simulink model "pardosealasim"  (R2023b)
settings: Solver=VariableStepAuto  StartTime=0.0  StopTime=12000  RelTol=1e-3
values from neighbouring files (symbols this model uses):
  A = [-(1/Tp) 1/Tp; Kp/(Kc*Tc) -((1+(Kp/Kc))/Tc)]    [pardoseala.m]
  B = [KE/(Kp*Tp) 0;0 1/Tc]    [pardoseala.m]
  C = [1 0;0 1]    [pardoseala.m]
  D = [0 0;0 0]    [pardoseala.m]
  Kc = 125    [pardoseala.m]
  KE = 1000    [pardoseala.m]
  Kp = 500    [pardoseala.m]
  Tc = 300    [pardoseala.m]
  Tp = 60    [pardoseala.m]
settings Model: Creator=Bianca  LastModifiedBy=Bianca

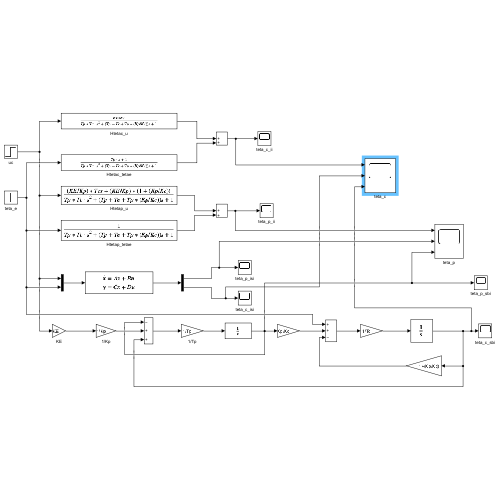
[thumbnail: Simulink's stored preview of the top-level diagram]
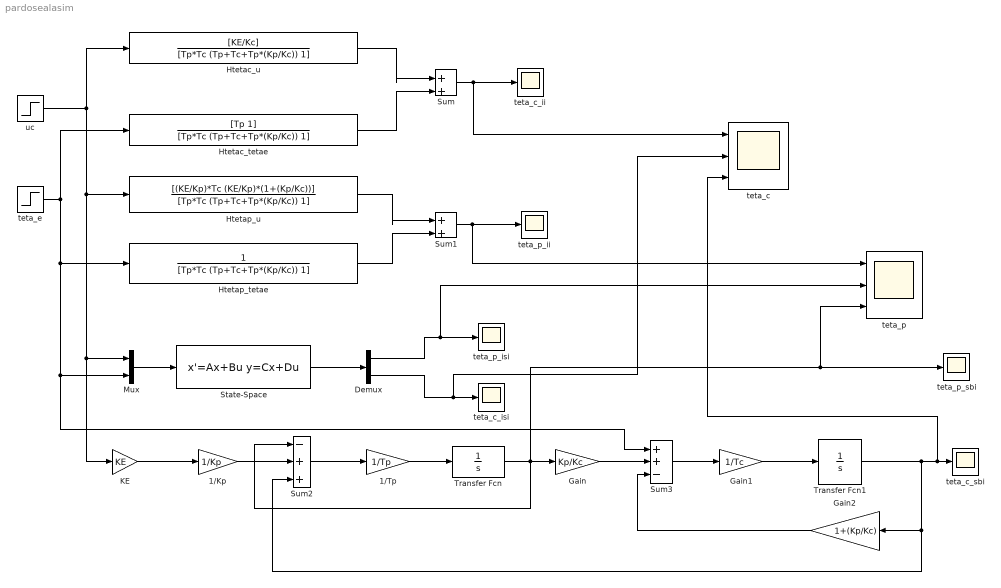
== system pardosealasim ==
  1/Kp : Gain  Gain=1/Kp
  1/Tp : Gain  Gain=1/Tp
  Demux : Demux  Outputs=2
  Gain : Gain  Gain=Kp/Kc
  Gain1 : Gain  Gain=1/Tc
  Gain2 : Gain  Gain=1+(Kp/Kc)
  Htetac_tetae : TransferFcn  Numerator=[Tp 1]  Denominator=[Tp*Tc (Tp+Tc+Tp*(Kp/Kc)) 1]
  Htetac_u : TransferFcn  Numerator=[KE/Kc]  Denominator=[Tp*Tc (Tp+Tc+Tp*(Kp/Kc)) 1]
  Htetap_tetae : TransferFcn  Denominator=[Tp*Tc (Tp+Tc+Tp*(Kp/Kc)) 1]
  Htetap_u : TransferFcn  Numerator=[(KE/Kp)*Tc (KE/Kp)*(1+(Kp/Kc))]  Denominator=[Tp*Tc (Tp+Tc+Tp*(Kp/Kc)) 1]
  KE : Gain  Gain=KE
  Mux : Mux  Inputs=2
  State-Space : StateSpace  A=A  B=B  C=C  D=D  InitialCondition=0
  Sum : Sum  Inputs=|++
  Sum1 : Sum  Inputs=|++
  Sum2 : Sum  Inputs=-++
  Sum3 : Sum  Inputs=++-
  Transfer Fcn : TransferFcn  Denominator=[1 0]
  Transfer Fcn1 : TransferFcn  Denominator=[1 0]
  teta_c : Scope  NumInputPorts=3
  teta_c_ii : Scope
  teta_c_isi : Scope
  teta_c_sbi : Scope
  teta_e : Step  Time=5000  After=-10  SampleTime=0
  teta_p : Scope  NumInputPorts=3
  teta_p_ii : Scope
  teta_p_isi : Scope
  teta_p_sbi : Scope
  uc : Step  Time=0  After=2.5  SampleTime=0
  wires:
  uc/1 -> KE/1, Mux/1, Htetap_u/1, Htetac_u/1
  teta_e/1 -> Htetac_tetae/1, Sum3/1, Mux/2, Htetap_tetae/1
  Htetac_u/1 -> Sum/1
  Htetac_tetae/1 -> Sum/2
  Htetap_u/1 -> Sum1/1
  Htetap_tetae/1 -> Sum1/2
  Sum/1 -> teta_c/1, teta_c_ii/1
  Sum1/1 -> teta_p/1, teta_p_ii/1
  Mux/1 -> State-Space/1
  State-Space/1 -> Demux/1
  Demux/1 -> teta_p/2, teta_p_isi/1
  Demux/2 -> teta_c/2, teta_c_isi/1
  KE/1 -> 1/Kp/1
  1/Kp/1 -> Sum2/2
  Sum2/1 -> 1/Tp/1
  1/Tp/1 -> Transfer Fcn/1
  Transfer Fcn/1 -> Sum2/1, teta_p/3, teta_p_sbi/1, Gain/1
  Gain/1 -> Sum3/2
  Sum3/1 -> Gain1/1
  Gain1/1 -> Transfer Fcn1/1
  Gain2/1 -> Sum3/3
  Transfer Fcn1/1 -> Sum2/3, Gain2/1, teta_c/3, teta_c_sbi/1
